simulink model "robot_2015"  (R2015b)
settings: Solver=VariableStepAuto  SolverMode=SingleTasking  StartTime=0.0  StopTime=10.0  RelTol=1e-3
model workspace: external: MATLAB File D:\Projects\SERTS\Body\v5.0\Matlab\Robot\robot_DataFile.m (data not in the file)
undefined symbols (not defined in the file or in its folder): smiData, X, Y, Z
libraries: sm_lib x7957, nesl_utility x37, simulink x36
(part 148 of 148)

== matlab function robot_2015/Leg_model_right_2/rightLegController /Subsystem/MATLAB Function1 ==
  data: kp input; kv input; x_desired input; dx_desired input; F input; T1 output; q1 input; q2 input; q3 input; x input; dx input; T2 output; T3 output
function [T1, T2, T3] = rightLegControl(kp, kv, x_desired, dx_desired, F, q1, q2, q3, x, dx)

g = [0     ;
     -9.8;
     0     ];

Mass_1 = [1.13997,  0,        0;
          0,        1.13997,  0;
          0,        0,        1.13997];

Iner_1 = [ 4695654.71e-09,      -3171848.05e-09,     212.52e-09;
           -3171848.05e-09,     4943364.65e-09,      -363.95e-09;
           212.52e-09,          -363.95e-09,         8566375.52e-09];

      
Mass_2 = [1.13649,  0,        0;
          0,        1.13649,  0;
          0,        0,        1.13649];

Iner_2 = [2554474.68e-09,      -231.05e-09,         -2855264.81e-09;
          -231.05e-09,         12519194.41e-09,     8.54e-09;
          -2855264.81e-09,     8.54e-09,            10576743.61e-09];

      
Mass_3 = [0.63820,  0,        0;
          0,        0.63820,  0;
          0,        0,        0.63280];
  
Iner_3 = [728680.81e-09,      -172.39e-09,        158.48e-09;
          -172.39e-09,        2618699.35e-09,     -3.33e-09;
          158.48e-09,         -3.33e-09,          2391085.66e-09];

      
Jv1 = [0.05737*cos(q1)-0.05549*sin(q1),    0, 0;
       0.05737*sin(q1)+0.05549*cos(q1),    0, 0;
       0,                                  0, 0];

Jw1 = [0, 0, 0;
       0, 0, 0;
       1, 0, 0];

   
Jv2 = [-0.09947*sin(q1)*cos(q2)+0.08747*cos(q1)-0.1225*sin(q1),  -0.09947*cos(q1)*sin(q2),      0;
       0.09947*cos(q1)*cos(q2)+0.08747*sin(q1)+0.1225*cos(q1),   -0.09947*sin(q1)*sin(q2),      0; 
       0,                                                        -0.09947*cos(q2),              0]; 
      
Jw2 = [0, -1, 0; 
       0,  0, 0; 
       1,  0, 0];
 
   
Jv3 = [-0.02559*sin(q1)*cos(q2-q3)-0.2*sin(q1)*cos(q2)-0.1225*sin(q1)+0.0525*cos(q1),  -0.02559*cos(q1)*sin(q2-q3)-0.2*cos(q1)*sin(q2),  0.02559*cos(q1)*sin(q2-q3);
       0.02559*cos(q1)*cos(q2-q3)+0.2*cos(q1)*cos(q2)+0.1225*cos(q1)+0.0525*sin(q1),   -0.02559*sin(q1)*sin(q2-q3)-0.2*sin(q1)*sin(q2),  0.02559*sin(q1)*sin(q2-q3);
       0,                                                                              -0.02559*cos(q2-q3)-0.2*cos(q2),                  0.02559*cos(q2-q3)       ];
      
Jw3 = [0, -1, 1;
       0,  0, 0;
       1,  0, 0];

   
JvEE = [-0.245*sin(q1)*cos(q2-q3)-0.2*sin(q1)*cos(q2)-0.1225*sin(q1)+0.0525*cos(q1),  -0.245*cos(q1)*sin(q2-q3)-0.2*cos(q1)*sin(q2),  0.245*cos(q1)*sin(q2-q3);
        0.245*cos(q1)*cos(q2-q3)+0.2*cos(q1)*cos(q2)+0.1225*cos(q1)+0.0525*sin(q1),   -0.245*sin(q1)*sin(q2-q3)-0.2*sin(q1)*sin(q2),  0.245*sin(q1)*sin(q2-q3);
        0,                                                                            -0.245*cos(q2-q3)-0.2*cos(q2),                  0.245*cos(q2-q3)       ];
   

Mass_q = Jv1'*Mass_1*Jv1 + Jw1'*Iner_1*Jw1 + Jv2'*Mass_2*Jv2 + Jw2'*Iner_2*Jw2 + Jv3'*Mass_3*Jv3 + Jw3'*Iner_3*Jw3;

Mass_x = JvEE'*pinv(JvEE*(inv(Mass_q))*JvEE');

Grav = Jv1'*Mass_1*g + Jv2'*Mass_2*g + Jv3'*Mass_3*g;

Force = JvEE'*F;

torque = Mass_x*((kp*(x_desired - x)) + (kv*(dx_desired - dx))) + Grav;

T1 = torque(1);
T2 = torque(2);
T3 = torque(3);

== matlab function robot_2015/Leg_model_right_2/rightLegController /Subsystem/MATLAB Function4 ==
  data: q1 input; x output; q2 input; q3 input
function x = Kinematics(q1, q2, q3)

leg = [0.245;
       0;
       0;
       1];
   
Trans0_3 = [cos(q1)*cos(q2-q3),    cos(q1)*sin(q2-q3),    sin(q1),       0.2*cos(q1)*cos(q2)+0.1225*cos(q1)+0.0525*sin(q1);
            sin(q1)*cos(q2-q3),    sin(q1)*sin(q2-q3),    -cos(q1),      0.2*sin(q1)*cos(q2)+0.1225*sin(q1)-0.0525*cos(q1);
            -sin(q2-q3),           cos(q2-q3),            0,             -0.2*sin(q2);
            0,                      0,                    0,              1];
        
x_temp = Trans0_3*leg;

x = x_temp(1:3);

== matlab function robot_2015/Leg_model_right_2/rightLegController /Subsystem/MATLAB Function5 ==
  data: q1 input; dx output; q2 input; q3 input; dq1 input; dq2 input; dq3 input
function dx = Jacobian(q1, q2, q3, dq1, dq2, dq3)

dq = [ dq1;
       dq2;
       dq3];

JvEE = [-0.245*sin(q1)*cos(q2-q3)-0.2*sin(q1)*cos(q2)-0.1225*sin(q1)+0.0525*cos(q1),  -0.245*cos(q1)*sin(q2-q3)-0.2*cos(q1)*sin(q2),  0.245*cos(q1)*sin(q2-q3);
        0.245*cos(q1)*cos(q2-q3)+0.2*cos(q1)*cos(q2)+0.1225*cos(q1)+0.0525*sin(q1),   -0.245*sin(q1)*sin(q2-q3)-0.2*sin(q1)*sin(q2),  0.245*sin(q1)*sin(q2-q3);
        0,                                                                            -0.245*cos(q2-q3)-0.2*cos(q2),                  0.245*cos(q2-q3)       ];
   
dx = JvEE*dq;

== matlab function robot_2015/Leg_model_left_2/leftLegController /MATLAB Function ==
  data: in1 input; out output; in2 input; in3 input
function out = matrix(in1, in2, in3)
out = [in1; in2; in3];

== matlab function robot_2015/Leg_model_left_2/leftLegController /MATLAB Function1 ==
  data: in1 input; out output; in2 input; in3 input
function out = matrix(in1, in2, in3)
out = [in1; in2; in3];

== matlab function robot_2015/Leg_model_left_2/leftLegController /MATLAB Function2 ==
  data: in1 input; out output; in2 input; in3 input
function out = matrix(in1, in2, in3)
out = [in1; in2; in3];

== matlab function robot_2015/Leg_model_left_2/leftLegController /Subsystem/MATLAB Function1 ==
  data: kp input; kv input; x_desired input; dx_desired input; F input; T1 output; q1 input; q2 input; q3 input; x input; dx input; T2 output; T3 output
function [T1, T2, T3] = rightLegControl(kp, kv, x_desired, dx_desired, F, q1, q2, q3, x, dx)

g = [0     ;
     -9.8;
     0     ];

Mass_1 = [1.13997,  0,        0;
          0,        1.13997,  0;
          0,        0,        1.13997];

Iner_1 = [ 4695654.71e-09,      3172004.63e-09,     -301.13e-09;
           3172004.63e-09,     4943364.65e-09,      -447.90e-09;
           -301.13e-09,          -447.90e-09,         8566375.52e-09];

      
Mass_2 = [1.13649,  0,        0;
          0,        1.13649,  0;
          0,        0,        1.13649];

Iner_2 = [2554474.68e-09,      35.35e-09,           2855264.81e-09;
          35.35e-09,           12519194.41e-09,     -51.54e-09;
          2855264.81e-09,     -51.54e-09,           10576743.61e-09];

      
Mass_3 = [0.63820,  0,        0;
          0,        0.63820,  0;
          0,        0,        0.63280];
  
Iner_3 = [728680.81e-09,      -172.39e-09,        158.48e-09;
          -172.39e-09,        2618699.35e-09,     -3.33e-09;
          158.48e-09,         -3.33e-09,          2391085.66e-09];

      
Jv1 = [-0.05737*cos(q1)-0.05549*sin(q1),    0, 0;
       -0.05737*sin(q1)+0.05549*cos(q1),    0, 0;
       0,                                  0, 0];

Jw1 = [0, 0, 0;
       0, 0, 0;
       1, 0, 0];

   
Jv2 = [-0.09947*sin(q1)*cos(q2)-0.08747*cos(q1)-0.1225*sin(q1),  -0.09947*cos(q1)*sin(q2),      0;
       0.09947*cos(q1)*cos(q2)-0.08747*sin(q1)+0.1225*cos(q1),   -0.09947*sin(q1)*sin(q2),      0; 
       0,                                                        -0.09947*cos(q2),              0]; 
      
Jw2 = [0, -1, 0; 
       0,  0, 0; 
       1,  0, 0];
 
   
Jv3 = [-0.02559*sin(q1)*cos(q2-q3)-0.2*sin(q1)*cos(q2)-0.1225*sin(q1)-0.0525*cos(q1),  -0.02559*cos(q1)*sin(q2-q3)-0.2*cos(q1)*sin(q2),  0.02559*cos(q1)*sin(q2-q3);
       0.02559*cos(q1)*cos(q2-q3)+0.2*cos(q1)*cos(q2)+0.1225*cos(q1)-0.0525*sin(q1),   -0.02559*sin(q1)*sin(q2-q3)-0.2*sin(q1)*sin(q2),  0.02559*sin(q1)*sin(q2-q3);
       0,                                                                              -0.02559*cos(q2-q3)-0.2*cos(q2),                  0.02559*cos(q2-q3)       ];
      
Jw3 = [0, -1, 1;
       0,  0, 0;
       1,  0, 0];

   
JvEE = [-0.245*sin(q1)*cos(q2-q3)-0.2*sin(q1)*cos(q2)-0.1225*sin(q1)-0.0525*cos(q1),  -0.245*cos(q1)*sin(q2-q3)-0.2*cos(q1)*sin(q2),  0.245*cos(q1)*sin(q2-q3);
        0.245*cos(q1)*cos(q2-q3)+0.2*cos(q1)*cos(q2)+0.1225*cos(q1)-0.0525*sin(q1),   -0.245*sin(q1)*sin(q2-q3)-0.2*sin(q1)*sin(q2),  0.245*sin(q1)*sin(q2-q3);
        0,                                                                            -0.245*cos(q2-q3)-0.2*cos(q2),                  0.245*cos(q2-q3)       ];
   

Mass_q = Jv1'*Mass_1*Jv1 + Jw1'*Iner_1*Jw1 + Jv2'*Mass_2*Jv2 + Jw2'*Iner_2*Jw2 + Jv3'*Mass_3*Jv3 + Jw3'*Iner_3*Jw3;

Mass_x = JvEE'*pinv(JvEE*(inv(Mass_q))*JvEE');

Grav = Jv1'*Mass_1*g + Jv2'*Mass_2*g + Jv3'*Mass_3*g;

Force = JvEE'*F;

torque = Mass_x*((kp*(x_desired - x)) + (kv*(dx_desired - dx))) + Grav;

T1 = torque(1);
T2 = torque(2);
T3 = torque(3);

== matlab function robot_2015/Leg_model_left_2/leftLegController /Subsystem/MATLAB Function4 ==
  data: q1 input; x output; q2 input; q3 input
function x = Kinematics(q1, q2, q3)

leg = [0.245;
       0;
       0;
       1];
   
Trans0_3 = [cos(q1)*cos(q2-q3),    cos(q1)*sin(q2-q3),    sin(q1),       0.2*cos(q1)*cos(q2)+0.1225*cos(q1)-0.0525*sin(q1);
            sin(q1)*cos(q2-q3),    sin(q1)*sin(q2-q3),    -cos(q1),      0.2*sin(q1)*cos(q2)+0.1225*sin(q1)+0.0525*cos(q1);
            -sin(q2-q3),           cos(q2-q3),            0,             -0.2*sin(q2);
            0,                      0,                    0,              1];
        
x_temp = Trans0_3*leg;

x = x_temp(1:3);

== matlab function robot_2015/Leg_model_left_2/leftLegController /Subsystem/MATLAB Function5 ==
  data: q1 input; dx output; q2 input; q3 input; dq1 input; dq2 input; dq3 input
function dx = Jacobian(q1, q2, q3, dq1, dq2, dq3)

dq = [ dq1;
       dq2;
       dq3];

JvEE = [-0.245*sin(q1)*cos(q2-q3)-0.2*sin(q1)*cos(q2)-0.1225*sin(q1)-0.0525*cos(q1),  -0.245*cos(q1)*sin(q2-q3)-0.2*cos(q1)*sin(q2),  0.245*cos(q1)*sin(q2-q3);
        0.245*cos(q1)*cos(q2-q3)+0.2*cos(q1)*cos(q2)+0.1225*cos(q1)-0.0525*sin(q1),   -0.245*sin(q1)*sin(q2-q3)-0.2*sin(q1)*sin(q2),  0.245*sin(q1)*sin(q2-q3);
        0,                                                                            -0.245*cos(q2-q3)-0.2*cos(q2),                  0.245*cos(q2-q3)       ];
   
dx = JvEE*dq;
